simulink model "lunar_lander_sim_PWPF_2023a"  (R2023a)
settings: Solver=FixedStepAuto  StartTime=0  StopTime=250  FixedStep=0.001  RelTol=1e-3
values from neighbouring files (symbols this model uses):
  D = 0:0.01:0.9    [limit_cycle_est.m]
undefined symbols (not defined in the file or in its folder): aMode
libraries: simulink_extras x8, slpidlib x6, shared6dofsys x2, sharedutil x2
settings Model: Creator=cnsl  LastModifiedBy=s3928

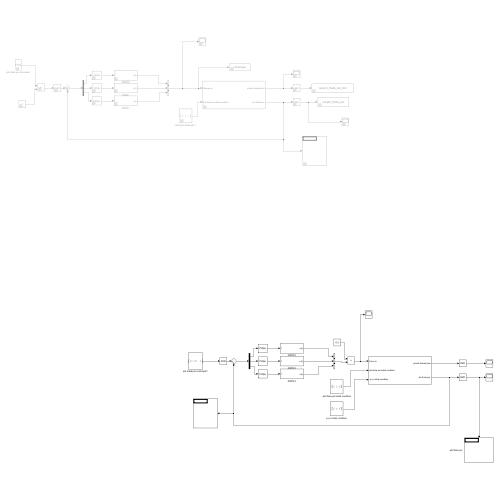
[thumbnail: Simulink's stored preview of the top-level diagram]
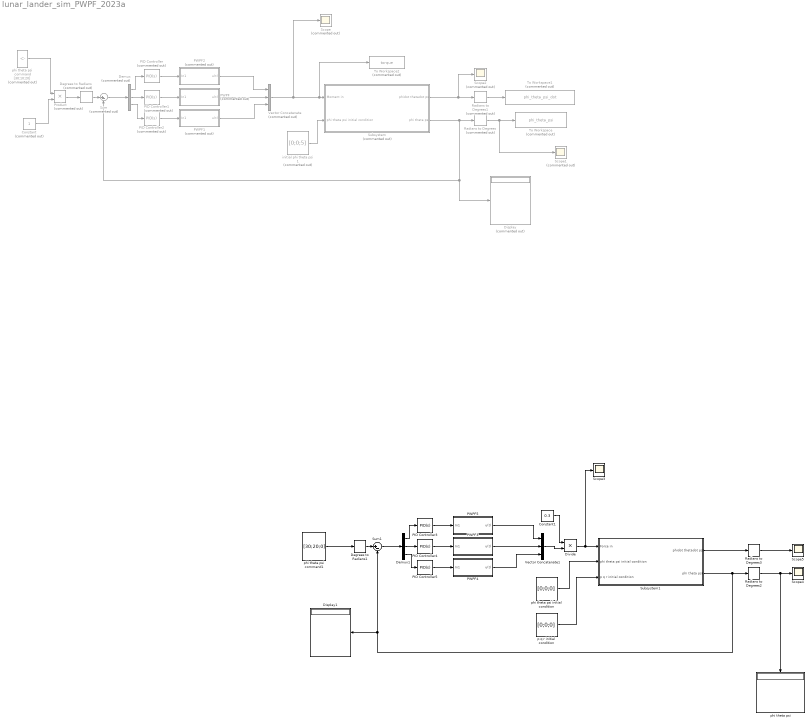
== system lunar_lander_sim_PWPF_2023a ==
  " phi theta psi initial condition" : Constant  Value=[0;0;0]
  Constant : Constant  Commented=on
  Constant1 : Constant  Value=0.3
  Degrees to Radians : simulink_extras/Transformations/Degrees to Radians  Commented=on
  Degrees to Radians1 : simulink_extras/Transformations/Degrees to Radians
  Demux : Demux  Commented=on  Outputs=3
  Demux1 : Demux  Outputs=3
  Display : Display  Commented=on
  Display1 : Display
  Divide : Product  Inputs=**
  PID Controller : slpidlib/PID Controller  Commented=on  Controller=PID  Form=Parallel  TimeDomain=Continuous-time  UseExternalTs=off  SampleTime=-1  IntegratorMethod=Forward Euler  FilterMethod=Forward Euler  ControllerParametersSource=internal  P=0  I=0  UseKiTs=off  D=0.602856201134272  N=5.45397025421619  UseFilter=on  TunerSelectOption=Transfer Function Based (PID Tuner App)  InitialConditionSource=internal  InitialConditionForIntegrator=0  InitialConditionForFilter=0  DifferentiatorICPrevScaledInput=0  ExternalReset=none  TrackingMode=off  Kt=1  LimitOutput=off  SatLimitsSource=internal  UpperSaturationLimit=inf  LowerSaturationLimit=-inf  LinearizeAsGain=on  AntiWindupMode=none  Kb=1  LimitIntegrator=off  UpperIntegratorSaturationLimit=inf  LowerIntegratorSaturationLimit=-inf  POutMin=[]  POutMax=[]  IOutMin=[]  IOutMax=[]  DOutMin=[]  DOutMax=[]  NOutMin=[]  NOutMax=[]  SumOutMin=[]  SumOutMax=[]  SaturationOutMin=[]  SaturationOutMax=[]  PParamMin=[]  PParamMax=[]  IParamMin=[]  IParamMax=[]  DParamMin=[]  DParamMax=[]  NParamMin=[]  NParamMax=[]  KbParamMin=[]  KbParamMax=[]  KtParamMin=[]  KtParamMax=[]  KbOutMin=[]  KbOutMax=[]  KtOutMin=[]  KtOutMax=[]  IntegratorOutMin=[]  IntegratorOutMax=[]  FilterOutMin=[]  FilterOutMax=[]  SumI1OutMin=[]  SumI1OutMax=[]  SumI2OutMin=[]  SumI2OutMax=[]  SumI3OutMin=[]  SumI3OutMax=[]  SumI4OutMin=[]  SumI4OutMax=[]  SumDOutMin=[]  SumDOutMax=[]  DifferentiatorOutMin=[]  DifferentiatorOutMax=[]  FilterDiffOutCoefMin=[]  FilterDiffOutCoefMax=[]  ReciprocalOutMin=[]  ReciprocalOutMax=[]  SumDenOutMin=[]  SumDenOutMax=[]  SumNumOutMin=[]  SumNumOutMax=[]  DivideOutMin=[]  DivideOutMax=[]  UdiffTsProdOutMin=[]  UdiffTsProdOutMax=[]  NTsProdOutMin=[]  NTsProdOutMax=[]  UintegralTsProdOutMin=[]  UintegralTsProdOutMax=[]  UngainTsProdOutMin=[]  UngainTsProdOutMax=[]  ClampingZeroOutDataTypeStr=Inherit: Inherit via back propagation  ClampingZeroOutMin=[]  ClampingZeroOutMax=[]  FilterDenConstantOutDataTypeStr=Inherit: Inherit via back propagation  FilterDenConstantOutMin=[]  FilterDenConstantOutMax=[]  PCopyOutDataTypeStr=Inherit: Inherit via back propagation  PCopyOutMin=[]  PCopyOutMax=[]  NCopyOutDataTypeStr=Inherit: Inherit via back propagation  NCopyOutMin=[]  NCopyOutMax=[]  IntegratorContinuousStateAttributes=''  IntegratorStateMustResolveToSignalObject=off  IntegratorRTWStateStorageClass=Auto  FilterContinuousStateAttributes=''  FilterStateMustResolveToSignalObject=off  FilterRTWStateStorageClass=Auto  ParallelPVariant=InternalParameters  IdealPVariant=Disabled  IVariant=InternalParameters  DVariant=InternalParameters  IntegratorVariant=Continuous  SatVariant=Disabled  AWVariant=Passthrough  PCopyVariant=Disabled  TRVariant=Disabled  FdbkBlocksVariant=Forward  IdealPFdbkVariant=Disabled  SatFdbkVariant=Disabled  DerivativeFilterVariant=ContFilter  NVariant=InternalParameters  NCopyVariant=Disabled  FilterICVariant=InternalICsFilter  IntegratorICVariant=InternalICs  ExternalResetVariant=Disabled  TRSumVariant=Passthrough  SumFdbkVariant=Disabled  SumVariant=Sum_PID  TsampFilterVariant=InternalTs  TsampNgainVariant=Passthrough  TsampIntegralVariant=Disabled_SignalSpec  ExternalSaturationOutDataTypeStr=Inherit: Same as second input
  PID Controller1 : slpidlib/PID Controller  Commented=on  Controller=PID  Form=Parallel  TimeDomain=Continuous-time  UseExternalTs=off  SampleTime=-1  IntegratorMethod=Forward Euler  FilterMethod=Forward Euler  ControllerParametersSource=internal  P=0.227642776770386  I=0  UseKiTs=off  D=1.19402712343922  N=5.45397025421619  UseFilter=on  TunerSelectOption=Transfer Function Based (PID Tuner App)  InitialConditionSource=internal  InitialConditionForIntegrator=0  InitialConditionForFilter=0  DifferentiatorICPrevScaledInput=0  ExternalReset=none  TrackingMode=off  Kt=1  LimitOutput=off  SatLimitsSource=internal  UpperSaturationLimit=inf  LowerSaturationLimit=-inf  LinearizeAsGain=on  AntiWindupMode=none  Kb=1  LimitIntegrator=off  UpperIntegratorSaturationLimit=inf  LowerIntegratorSaturationLimit=-inf  POutMin=[]  POutMax=[]  IOutMin=[]  IOutMax=[]  DOutMin=[]  DOutMax=[]  NOutMin=[]  NOutMax=[]  SumOutMin=[]  SumOutMax=[]  SaturationOutMin=[]  SaturationOutMax=[]  PParamMin=[]  PParamMax=[]  IParamMin=[]  IParamMax=[]  DParamMin=[]  DParamMax=[]  NParamMin=[]  NParamMax=[]  KbParamMin=[]  KbParamMax=[]  KtParamMin=[]  KtParamMax=[]  KbOutMin=[]  KbOutMax=[]  KtOutMin=[]  KtOutMax=[]  IntegratorOutMin=[]  IntegratorOutMax=[]  FilterOutMin=[]  FilterOutMax=[]  SumI1OutMin=[]  SumI1OutMax=[]  SumI2OutMin=[]  SumI2OutMax=[]  SumI3OutMin=[]  SumI3OutMax=[]  SumI4OutMin=[]  SumI4OutMax=[]  SumDOutMin=[]  SumDOutMax=[]  DifferentiatorOutMin=[]  DifferentiatorOutMax=[]  FilterDiffOutCoefMin=[]  FilterDiffOutCoefMax=[]  ReciprocalOutMin=[]  ReciprocalOutMax=[]  SumDenOutMin=[]  SumDenOutMax=[]  SumNumOutMin=[]  SumNumOutMax=[]  DivideOutMin=[]  DivideOutMax=[]  UdiffTsProdOutMin=[]  UdiffTsProdOutMax=[]  NTsProdOutMin=[]  NTsProdOutMax=[]  UintegralTsProdOutMin=[]  UintegralTsProdOutMax=[]  UngainTsProdOutMin=[]  UngainTsProdOutMax=[]  ClampingZeroOutDataTypeStr=Inherit: Inherit via back propagation  ClampingZeroOutMin=[]  ClampingZeroOutMax=[]  FilterDenConstantOutDataTypeStr=Inherit: Inherit via back propagation  FilterDenConstantOutMin=[]  FilterDenConstantOutMax=[]  PCopyOutDataTypeStr=Inherit: Inherit via back propagation  PCopyOutMin=[]  PCopyOutMax=[]  NCopyOutDataTypeStr=Inherit: Inherit via back propagation  NCopyOutMin=[]  NCopyOutMax=[]  IntegratorContinuousStateAttributes=''  IntegratorStateMustResolveToSignalObject=off  IntegratorRTWStateStorageClass=Auto  FilterContinuousStateAttributes=''  FilterStateMustResolveToSignalObject=off  FilterRTWStateStorageClass=Auto  ParallelPVariant=InternalParameters  IdealPVariant=Disabled  IVariant=InternalParameters  DVariant=InternalParameters  IntegratorVariant=Continuous  SatVariant=Disabled  AWVariant=Passthrough  PCopyVariant=Disabled  TRVariant=Disabled  FdbkBlocksVariant=Forward  IdealPFdbkVariant=Disabled  SatFdbkVariant=Disabled  DerivativeFilterVariant=ContFilter  NVariant=InternalParameters  NCopyVariant=Disabled  FilterICVariant=InternalICsFilter  IntegratorICVariant=InternalICs  ExternalResetVariant=Disabled  TRSumVariant=Passthrough  SumFdbkVariant=Disabled  SumVariant=Sum_PID  TsampFilterVariant=InternalTs  TsampNgainVariant=Passthrough  TsampIntegralVariant=Disabled_SignalSpec  ExternalSaturationOutDataTypeStr=Inherit: Same as second input
  PID Controller2 : slpidlib/PID Controller  Commented=on  Controller=PID  Form=Parallel  TimeDomain=Continuous-time  UseExternalTs=off  SampleTime=-1  IntegratorMethod=Forward Euler  FilterMethod=Forward Euler  ControllerParametersSource=internal  P=0.227642776770386  I=0  UseKiTs=off  D=1.19402712343922  N=5.45397025421619  UseFilter=on  TunerSelectOption=Transfer Function Based (PID Tuner App)  InitialConditionSource=internal  InitialConditionForIntegrator=0  InitialConditionForFilter=0  DifferentiatorICPrevScaledInput=0  ExternalReset=none  TrackingMode=off  Kt=1  LimitOutput=off  SatLimitsSource=internal  UpperSaturationLimit=inf  LowerSaturationLimit=-inf  LinearizeAsGain=on  AntiWindupMode=none  Kb=1  LimitIntegrator=off  UpperIntegratorSaturationLimit=inf  LowerIntegratorSaturationLimit=-inf  POutMin=[]  POutMax=[]  IOutMin=[]  IOutMax=[]  DOutMin=[]  DOutMax=[]  NOutMin=[]  NOutMax=[]  SumOutMin=[]  SumOutMax=[]  SaturationOutMin=[]  SaturationOutMax=[]  PParamMin=[]  PParamMax=[]  IParamMin=[]  IParamMax=[]  DParamMin=[]  DParamMax=[]  NParamMin=[]  NParamMax=[]  KbParamMin=[]  KbParamMax=[]  KtParamMin=[]  KtParamMax=[]  KbOutMin=[]  KbOutMax=[]  KtOutMin=[]  KtOutMax=[]  IntegratorOutMin=[]  IntegratorOutMax=[]  FilterOutMin=[]  FilterOutMax=[]  SumI1OutMin=[]  SumI1OutMax=[]  SumI2OutMin=[]  SumI2OutMax=[]  SumI3OutMin=[]  SumI3OutMax=[]  SumI4OutMin=[]  SumI4OutMax=[]  SumDOutMin=[]  SumDOutMax=[]  DifferentiatorOutMin=[]  DifferentiatorOutMax=[]  FilterDiffOutCoefMin=[]  FilterDiffOutCoefMax=[]  ReciprocalOutMin=[]  ReciprocalOutMax=[]  SumDenOutMin=[]  SumDenOutMax=[]  SumNumOutMin=[]  SumNumOutMax=[]  DivideOutMin=[]  DivideOutMax=[]  UdiffTsProdOutMin=[]  UdiffTsProdOutMax=[]  NTsProdOutMin=[]  NTsProdOutMax=[]  UintegralTsProdOutMin=[]  UintegralTsProdOutMax=[]  UngainTsProdOutMin=[]  UngainTsProdOutMax=[]  ClampingZeroOutDataTypeStr=Inherit: Inherit via back propagation  ClampingZeroOutMin=[]  ClampingZeroOutMax=[]  FilterDenConstantOutDataTypeStr=Inherit: Inherit via back propagation  FilterDenConstantOutMin=[]  FilterDenConstantOutMax=[]  PCopyOutDataTypeStr=Inherit: Inherit via back propagation  PCopyOutMin=[]  PCopyOutMax=[]  NCopyOutDataTypeStr=Inherit: Inherit via back propagation  NCopyOutMin=[]  NCopyOutMax=[]  IntegratorContinuousStateAttributes=''  IntegratorStateMustResolveToSignalObject=off  IntegratorRTWStateStorageClass=Auto  FilterContinuousStateAttributes=''  FilterStateMustResolveToSignalObject=off  FilterRTWStateStorageClass=Auto  ParallelPVariant=InternalParameters  IdealPVariant=Disabled  IVariant=InternalParameters  DVariant=InternalParameters  IntegratorVariant=Continuous  SatVariant=Disabled  AWVariant=Passthrough  PCopyVariant=Disabled  TRVariant=Disabled  FdbkBlocksVariant=Forward  IdealPFdbkVariant=Disabled  SatFdbkVariant=Disabled  DerivativeFilterVariant=ContFilter  NVariant=InternalParameters  NCopyVariant=Disabled  FilterICVariant=InternalICsFilter  IntegratorICVariant=InternalICs  ExternalResetVariant=Disabled  TRSumVariant=Passthrough  SumFdbkVariant=Disabled  SumVariant=Sum_PID  TsampFilterVariant=InternalTs  TsampNgainVariant=Passthrough  TsampIntegralVariant=Disabled_SignalSpec  ExternalSaturationOutDataTypeStr=Inherit: Same as second input
  PID Controller3 : slpidlib/PID Controller  Controller=PID  Form=Parallel  TimeDomain=Continuous-time  UseExternalTs=off  SampleTime=-1  IntegratorMethod=Forward Euler  FilterMethod=Forward Euler  ControllerParametersSource=internal  P=3  I=0.5  UseKiTs=off  D=8  N=1000  UseFilter=on  TunerSelectOption=Transfer Function Based (PID Tuner App)  InitialConditionSource=internal  InitialConditionForIntegrator=0  InitialConditionForFilter=0  DifferentiatorICPrevScaledInput=0  ExternalReset=none  TrackingMode=off  Kt=1  LimitOutput=off  SatLimitsSource=internal  UpperSaturationLimit=inf  LowerSaturationLimit=-inf  LinearizeAsGain=on  AntiWindupMode=none  Kb=1  LimitIntegrator=off  UpperIntegratorSaturationLimit=inf  LowerIntegratorSaturationLimit=-inf  POutMin=[]  POutMax=[]  IOutMin=[]  IOutMax=[]  DOutMin=[]  DOutMax=[]  NOutMin=[]  NOutMax=[]  SumOutMin=[]  SumOutMax=[]  SaturationOutMin=[]  SaturationOutMax=[]  PParamMin=[]  PParamMax=[]  IParamMin=[]  IParamMax=[]  DParamMin=[]  DParamMax=[]  NParamMin=[]  NParamMax=[]  KbParamMin=[]  KbParamMax=[]  KtParamMin=[]  KtParamMax=[]  KbOutMin=[]  KbOutMax=[]  KtOutMin=[]  KtOutMax=[]  IntegratorOutMin=[]  IntegratorOutMax=[]  FilterOutMin=[]  FilterOutMax=[]  SumI1OutMin=[]  SumI1OutMax=[]  SumI2OutMin=[]  SumI2OutMax=[]  SumI3OutMin=[]  SumI3OutMax=[]  SumI4OutMin=[]  SumI4OutMax=[]  SumDOutMin=[]  SumDOutMax=[]  DifferentiatorOutMin=[]  DifferentiatorOutMax=[]  FilterDiffOutCoefMin=[]  FilterDiffOutCoefMax=[]  ReciprocalOutMin=[]  ReciprocalOutMax=[]  SumDenOutMin=[]  SumDenOutMax=[]  SumNumOutMin=[]  SumNumOutMax=[]  DivideOutMin=[]  DivideOutMax=[]  UdiffTsProdOutMin=[]  UdiffTsProdOutMax=[]  NTsProdOutMin=[]  NTsProdOutMax=[]  UintegralTsProdOutMin=[]  UintegralTsProdOutMax=[]  UngainTsProdOutMin=[]  UngainTsProdOutMax=[]  ClampingZeroOutDataTypeStr=Inherit: Inherit via back propagation  ClampingZeroOutMin=[]  ClampingZeroOutMax=[]  FilterDenConstantOutDataTypeStr=Inherit: Inherit via back propagation  FilterDenConstantOutMin=[]  FilterDenConstantOutMax=[]  PCopyOutDataTypeStr=Inherit: Inherit via back propagation  PCopyOutMin=[]  PCopyOutMax=[]  NCopyOutDataTypeStr=Inherit: Inherit via back propagation  NCopyOutMin=[]  NCopyOutMax=[]  IntegratorContinuousStateAttributes=''  IntegratorStateMustResolveToSignalObject=off  IntegratorRTWStateStorageClass=Auto  FilterContinuousStateAttributes=''  FilterStateMustResolveToSignalObject=off  FilterRTWStateStorageClass=Auto  ParallelPVariant=InternalParameters  IdealPVariant=Disabled  IVariant=InternalParameters  DVariant=InternalParameters  IntegratorVariant=Continuous  SatVariant=Disabled  AWVariant=Passthrough  PCopyVariant=Disabled  TRVariant=Disabled  FdbkBlocksVariant=Forward  IdealPFdbkVariant=Disabled  SatFdbkVariant=Disabled  DerivativeFilterVariant=ContFilter  NVariant=InternalParameters  NCopyVariant=Disabled  FilterICVariant=InternalICsFilter  IntegratorICVariant=InternalICs  ExternalResetVariant=Disabled  TRSumVariant=Passthrough  SumFdbkVariant=Disabled  SumVariant=Sum_PID  TsampFilterVariant=InternalTs  TsampNgainVariant=Passthrough  TsampIntegralVariant=Disabled_SignalSpec  ExternalSaturationOutDataTypeStr=Inherit: Same as second input
  PID Controller4 : slpidlib/PID Controller  Controller=PID  Form=Parallel  TimeDomain=Continuous-time  UseExternalTs=off  SampleTime=-1  IntegratorMethod=Forward Euler  FilterMethod=Forward Euler  ControllerParametersSource=internal  P=2  I=0.1  UseKiTs=off  D=8  N=1000  UseFilter=on  TunerSelectOption=Transfer Function Based (PID Tuner App)  InitialConditionSource=internal  InitialConditionForIntegrator=0  InitialConditionForFilter=0  DifferentiatorICPrevScaledInput=0  ExternalReset=none  TrackingMode=off  Kt=1  LimitOutput=off  SatLimitsSource=internal  UpperSaturationLimit=inf  LowerSaturationLimit=-inf  LinearizeAsGain=on  AntiWindupMode=none  Kb=1  LimitIntegrator=off  UpperIntegratorSaturationLimit=inf  LowerIntegratorSaturationLimit=-inf  POutMin=[]  POutMax=[]  IOutMin=[]  IOutMax=[]  DOutMin=[]  DOutMax=[]  NOutMin=[]  NOutMax=[]  SumOutMin=[]  SumOutMax=[]  SaturationOutMin=[]  SaturationOutMax=[]  PParamMin=[]  PParamMax=[]  IParamMin=[]  IParamMax=[]  DParamMin=[]  DParamMax=[]  NParamMin=[]  NParamMax=[]  KbParamMin=[]  KbParamMax=[]  KtParamMin=[]  KtParamMax=[]  KbOutMin=[]  KbOutMax=[]  KtOutMin=[]  KtOutMax=[]  IntegratorOutMin=[]  IntegratorOutMax=[]  FilterOutMin=[]  FilterOutMax=[]  SumI1OutMin=[]  SumI1OutMax=[]  SumI2OutMin=[]  SumI2OutMax=[]  SumI3OutMin=[]  SumI3OutMax=[]  SumI4OutMin=[]  SumI4OutMax=[]  SumDOutMin=[]  SumDOutMax=[]  DifferentiatorOutMin=[]  DifferentiatorOutMax=[]  FilterDiffOutCoefMin=[]  FilterDiffOutCoefMax=[]  ReciprocalOutMin=[]  ReciprocalOutMax=[]  SumDenOutMin=[]  SumDenOutMax=[]  SumNumOutMin=[]  SumNumOutMax=[]  DivideOutMin=[]  DivideOutMax=[]  UdiffTsProdOutMin=[]  UdiffTsProdOutMax=[]  NTsProdOutMin=[]  NTsProdOutMax=[]  UintegralTsProdOutMin=[]  UintegralTsProdOutMax=[]  UngainTsProdOutMin=[]  UngainTsProdOutMax=[]  ClampingZeroOutDataTypeStr=Inherit: Inherit via back propagation  ClampingZeroOutMin=[]  ClampingZeroOutMax=[]  FilterDenConstantOutDataTypeStr=Inherit: Inherit via back propagation  FilterDenConstantOutMin=[]  FilterDenConstantOutMax=[]  PCopyOutDataTypeStr=Inherit: Inherit via back propagation  PCopyOutMin=[]  PCopyOutMax=[]  NCopyOutDataTypeStr=Inherit: Inherit via back propagation  NCopyOutMin=[]  NCopyOutMax=[]  IntegratorContinuousStateAttributes=''  IntegratorStateMustResolveToSignalObject=off  IntegratorRTWStateStorageClass=Auto  FilterContinuousStateAttributes=''  FilterStateMustResolveToSignalObject=off  FilterRTWStateStorageClass=Auto  ParallelPVariant=InternalParameters  IdealPVariant=Disabled  IVariant=InternalParameters  DVariant=InternalParameters  IntegratorVariant=Continuous  SatVariant=Disabled  AWVariant=Passthrough  PCopyVariant=Disabled  TRVariant=Disabled  FdbkBlocksVariant=Forward  IdealPFdbkVariant=Disabled  SatFdbkVariant=Disabled  DerivativeFilterVariant=ContFilter  NVariant=InternalParameters  NCopyVariant=Disabled  FilterICVariant=InternalICsFilter  IntegratorICVariant=InternalICs  ExternalResetVariant=Disabled  TRSumVariant=Passthrough  SumFdbkVariant=Disabled  SumVariant=Sum_PID  TsampFilterVariant=InternalTs  TsampNgainVariant=Passthrough  TsampIntegralVariant=Disabled_SignalSpec  ExternalSaturationOutDataTypeStr=Inherit: Same as second input
  PID Controller5 : slpidlib/PID Controller  Controller=PID  Form=Parallel  TimeDomain=Continuous-time  UseExternalTs=off  SampleTime=-1  IntegratorMethod=Forward Euler  FilterMethod=Forward Euler  ControllerParametersSource=internal  P=3  I=0.2  UseKiTs=off  D=12  N=1000  UseFilter=on  TunerSelectOption=Transfer Function Based (PID Tuner App)  InitialConditionSource=internal  InitialConditionForIntegrator=0  InitialConditionForFilter=0  DifferentiatorICPrevScaledInput=0  ExternalReset=none  TrackingMode=off  Kt=1  LimitOutput=off  SatLimitsSource=internal  UpperSaturationLimit=inf  LowerSaturationLimit=-inf  LinearizeAsGain=on  AntiWindupMode=none  Kb=1  LimitIntegrator=off  UpperIntegratorSaturationLimit=inf  LowerIntegratorSaturationLimit=-inf  POutMin=[]  POutMax=[]  IOutMin=[]  IOutMax=[]  DOutMin=[]  DOutMax=[]  NOutMin=[]  NOutMax=[]  SumOutMin=[]  SumOutMax=[]  SaturationOutMin=[]  SaturationOutMax=[]  PParamMin=[]  PParamMax=[]  IParamMin=[]  IParamMax=[]  DParamMin=[]  DParamMax=[]  NParamMin=[]  NParamMax=[]  KbParamMin=[]  KbParamMax=[]  KtParamMin=[]  KtParamMax=[]  KbOutMin=[]  KbOutMax=[]  KtOutMin=[]  KtOutMax=[]  IntegratorOutMin=[]  IntegratorOutMax=[]  FilterOutMin=[]  FilterOutMax=[]  SumI1OutMin=[]  SumI1OutMax=[]  SumI2OutMin=[]  SumI2OutMax=[]  SumI3OutMin=[]  SumI3OutMax=[]  SumI4OutMin=[]  SumI4OutMax=[]  SumDOutMin=[]  SumDOutMax=[]  DifferentiatorOutMin=[]  DifferentiatorOutMax=[]  FilterDiffOutCoefMin=[]  FilterDiffOutCoefMax=[]  ReciprocalOutMin=[]  ReciprocalOutMax=[]  SumDenOutMin=[]  SumDenOutMax=[]  SumNumOutMin=[]  SumNumOutMax=[]  DivideOutMin=[]  DivideOutMax=[]  UdiffTsProdOutMin=[]  UdiffTsProdOutMax=[]  NTsProdOutMin=[]  NTsProdOutMax=[]  UintegralTsProdOutMin=[]  UintegralTsProdOutMax=[]  UngainTsProdOutMin=[]  UngainTsProdOutMax=[]  ClampingZeroOutDataTypeStr=Inherit: Inherit via back propagation  ClampingZeroOutMin=[]  ClampingZeroOutMax=[]  FilterDenConstantOutDataTypeStr=Inherit: Inherit via back propagation  FilterDenConstantOutMin=[]  FilterDenConstantOutMax=[]  PCopyOutDataTypeStr=Inherit: Inherit via back propagation  PCopyOutMin=[]  PCopyOutMax=[]  NCopyOutDataTypeStr=Inherit: Inherit via back propagation  NCopyOutMin=[]  NCopyOutMax=[]  IntegratorContinuousStateAttributes=''  IntegratorStateMustResolveToSignalObject=off  IntegratorRTWStateStorageClass=Auto  FilterContinuousStateAttributes=''  FilterStateMustResolveToSignalObject=off  FilterRTWStateStorageClass=Auto  ParallelPVariant=InternalParameters  IdealPVariant=Disabled  IVariant=InternalParameters  DVariant=InternalParameters  IntegratorVariant=Continuous  SatVariant=Disabled  AWVariant=Passthrough  PCopyVariant=Disabled  TRVariant=Disabled  FdbkBlocksVariant=Forward  IdealPFdbkVariant=Disabled  SatFdbkVariant=Disabled  DerivativeFilterVariant=ContFilter  NVariant=InternalParameters  NCopyVariant=Disabled  FilterICVariant=InternalICsFilter  IntegratorICVariant=InternalICs  ExternalResetVariant=Disabled  TRSumVariant=Passthrough  SumFdbkVariant=Disabled  SumVariant=Sum_PID  TsampFilterVariant=InternalTs  TsampNgainVariant=Passthrough  TsampIntegralVariant=Disabled_SignalSpec  ExternalSaturationOutDataTypeStr=Inherit: Same as second input
  PWPF : Subsystem  Commented=on
  PWPF1 : Subsystem  Commented=on
  PWPF2 : Subsystem  Commented=on
  PWPF3 : Subsystem
  PWPF4 : Subsystem
  PWPF5 : Subsystem
  Product : Product  Commented=on
  Radians to Degrees : simulink_extras/Transformations/Radians to Degrees  Commented=on
  Radians to Degrees1 : simulink_extras/Transformations/Radians to Degrees  Commented=on
  Radians to Degrees2 : simulink_extras/Transformations/Radians to Degrees
  Radians to Degrees3 : simulink_extras/Transformations/Radians to Degrees
  Scope : Scope  Commented=on
  Scope1 : Scope  Commented=on
  Scope2 : Scope  Commented=on
  Scope3 : Scope
  Scope4 : Scope
  Scope5 : Scope
  Subsystem : Subsystem  Commented=on
  Subsystem1 : Subsystem
  Sum : Sum  Commented=on  Inputs=|+-
  Sum1 : Sum  Inputs=|+-
  To Workspace : ToWorkspace  Commented=on  VariableName=phi_theta_psi  SaveFormat=Timeseries  SampleTime=-1
  To Workspace1 : ToWorkspace  Commented=on  VariableName=phi_theta_psi_dot  SaveFormat=Timeseries  SampleTime=-1
  To Workspace2 : ToWorkspace  Commented=on  VariableName=torque  SaveFormat=Timeseries  SampleTime=-1
  Vector Concatenate : Concatenate  Commented=on  NumInputs=3
  Vector Concatenate1 : Concatenate  NumInputs=3
  initial phi theta psi 1 : Constant  Commented=on  Value=[0;0;5]
  p q r initial condition : Constant  Value=[0;0;0]
  "phi theta psi " : Display
  phi theta psi command : Constant  Commented=on  Value=[30;10;20]
  phi theta psi command1 : Constant  Value=[30;20;0]
  wires:
  Subsystem/2("phi theta psi ") -> Radians to Degrees/1, Display/1, Sum/2
  Degrees to Radians/1 -> Sum/1
  Radians to Degrees/1 -> Scope1/1, To Workspace/1
  Vector Concatenate/1 -> Scope/1, Subsystem/1(Moment in), To Workspace2/1
  initial phi theta psi 1/1 -> Subsystem/2("phi theta psi initial condition ")
  phi theta psi command/1 -> Product/1
  Product/1 -> Degrees to Radians/1
  Constant/1 -> Product/2
  Demux/1 -> PID Controller/1
  Demux/3 -> PID Controller2/1
  PID Controller2/1 -> PWPF1/1(In1)
  Subsystem/1(phidot thetadot psi) -> Scope2/1, Radians to Degrees1/1
  Sum/1 -> Demux/1
  Radians to Degrees1/1 -> To Workspace1/1
  PID Controller/1 -> PWPF2/1(In1)
  Demux/2 -> PID Controller1/1
  PWPF/1(u(t)) -> Vector Concatenate/2
  PID Controller1/1 -> PWPF/1(In1)
  PWPF1/1(u(t)) -> Vector Concatenate/3
  PWPF2/1(u(t)) -> Vector Concatenate/1
  Sum1/1 -> Demux1/1
  phi theta psi command1/1 -> Degrees to Radians1/1
  Demux1/2 -> PID Controller4/1
  Demux1/3 -> PID Controller5/1
  Subsystem1/1(phidot thetadot psi) -> Radians to Degrees3/1
  Demux1/1 -> PID Controller3/1
  Degrees to Radians1/1 -> Sum1/1
  Radians to Degrees2/1 -> Scope4/1, "phi theta psi "/1
  " phi theta psi initial condition"/1 -> Subsystem1/2("phi theta psi initial condition ")
  Subsystem1/2("phi theta psi ") -> Radians to Degrees2/1, Sum1/2, Display1/1
  PID Controller3/1 -> PWPF5/1(In1)
  PID Controller5/1 -> PWPF4/1(In1)
  PID Controller4/1 -> PWPF3/1(In1)
  Radians to Degrees3/1 -> Scope5/1
  p q r initial condition/1 -> Subsystem1/3(" p q r initial condition")
  PWPF3/1(u(t)) -> Vector Concatenate1/2
  PWPF4/1(u(t)) -> Vector Concatenate1/3
  PWPF5/1(u(t)) -> Vector Concatenate1/1
  Vector Concatenate1/1 -> Divide/2
  Divide/1 -> Scope3/1, Subsystem1/1(Force in)
  Constant1/1 -> Divide/1

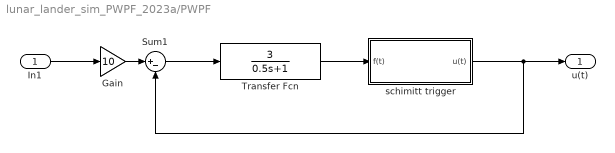
== system lunar_lander_sim_PWPF_2023a/PWPF ==
  In1 : Inport
  Gain : Gain  Gain=10
  Sum1 : Sum  Inputs=|+-
  Transfer Fcn : TransferFcn  Numerator=[3]  Denominator=[0.5 1]
  schimitt trigger : Subsystem
  u(t) : Outport
  wires:
  schimitt trigger/1(u(t)) -> u(t)/1, Sum1/2
  Gain/1 -> Sum1/1
  Sum1/1 -> Transfer Fcn/1
  Transfer Fcn/1 -> schimitt trigger/1(f(t))
  In1/1 -> Gain/1

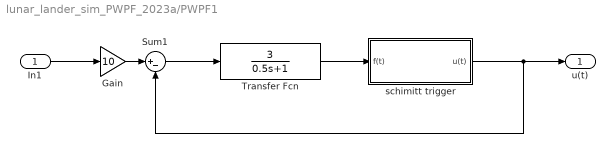
== system lunar_lander_sim_PWPF_2023a/PWPF1 ==
  In1 : Inport
  Gain : Gain  Gain=10
  Sum1 : Sum  Inputs=|+-
  Transfer Fcn : TransferFcn  Numerator=[3]  Denominator=[0.5 1]
  schimitt trigger : Subsystem
  u(t) : Outport
  wires:
  In1/1 -> Gain/1
  Transfer Fcn/1 -> schimitt trigger/1(f(t))
  Sum1/1 -> Transfer Fcn/1
  Gain/1 -> Sum1/1
  schimitt trigger/1(u(t)) -> Sum1/2, u(t)/1

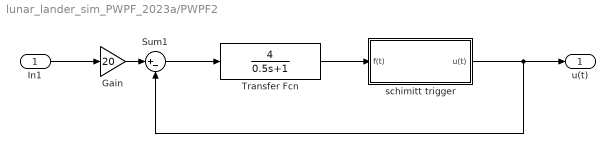
== system lunar_lander_sim_PWPF_2023a/PWPF2 ==
  In1 : Inport
  Gain : Gain  Gain=20
  Sum1 : Sum  Inputs=|+-
  Transfer Fcn : TransferFcn  Numerator=[4]  Denominator=[0.5 1]
  schimitt trigger : Subsystem
  u(t) : Outport
  wires:
  schimitt trigger/1(u(t)) -> u(t)/1, Sum1/2
  Gain/1 -> Sum1/1
  Sum1/1 -> Transfer Fcn/1
  Transfer Fcn/1 -> schimitt trigger/1(f(t))
  In1/1 -> Gain/1

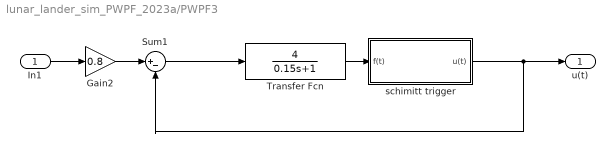
== system lunar_lander_sim_PWPF_2023a/PWPF3 ==
  In1 : Inport
  Gain2 : Gain  Gain=0.8
  Sum1 : Sum  Inputs=|+-
  Transfer Fcn : TransferFcn  Numerator=[4]  Denominator=[0.15 1]
  schimitt trigger : Subsystem
  u(t) : Outport
  wires:
  In1/1 -> Gain2/1
  Gain2/1 -> Sum1/1
  schimitt trigger/1(u(t)) -> u(t)/1, Sum1/2
  Sum1/1 -> Transfer Fcn/1
  Transfer Fcn/1 -> schimitt trigger/1(f(t))

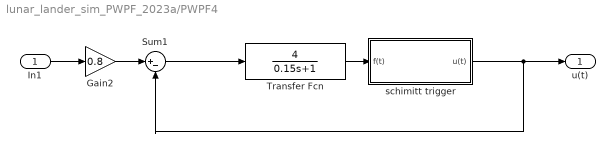
== system lunar_lander_sim_PWPF_2023a/PWPF4 ==
  In1 : Inport
  Gain2 : Gain  Gain=0.8
  Sum1 : Sum  Inputs=|+-
  Transfer Fcn : TransferFcn  Numerator=[4]  Denominator=[0.15 1]
  schimitt trigger : Subsystem
  u(t) : Outport
  wires:
  Transfer Fcn/1 -> schimitt trigger/1(f(t))
  Sum1/1 -> Transfer Fcn/1
  schimitt trigger/1(u(t)) -> Sum1/2, u(t)/1
  Gain2/1 -> Sum1/1
  In1/1 -> Gain2/1

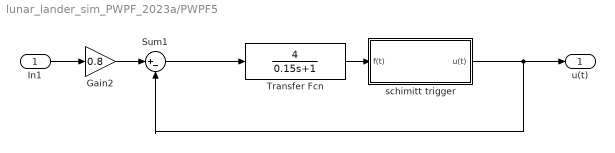
== system lunar_lander_sim_PWPF_2023a/PWPF5 ==
  In1 : Inport
  Gain2 : Gain  Gain=0.8
  Sum1 : Sum  Inputs=|+-
  Transfer Fcn : TransferFcn  Numerator=[4]  Denominator=[0.15 1]
  schimitt trigger : Subsystem
  u(t) : Outport
  wires:
  Transfer Fcn/1 -> schimitt trigger/1(f(t))
  Sum1/1 -> Transfer Fcn/1
  schimitt trigger/1(u(t)) -> Sum1/2, u(t)/1
  Gain2/1 -> Sum1/1
  In1/1 -> Gain2/1

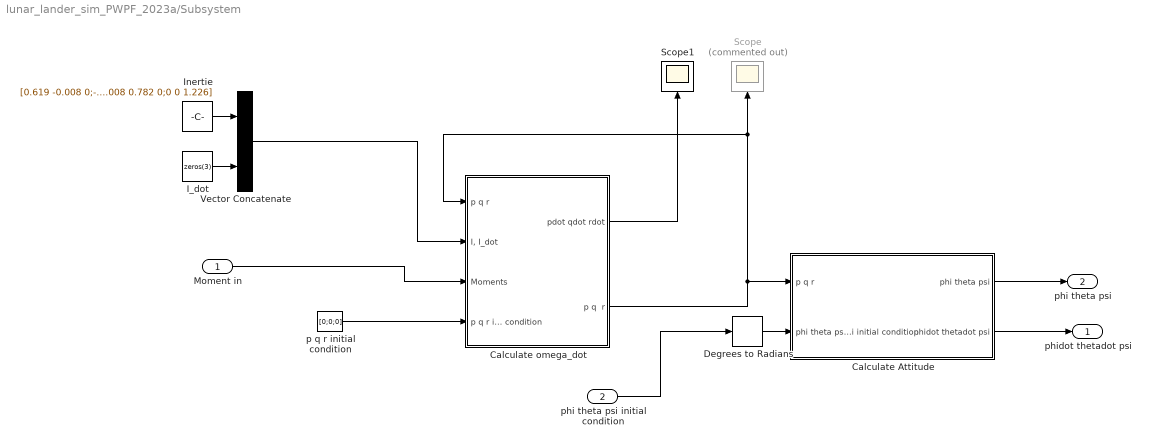
== system lunar_lander_sim_PWPF_2023a/Subsystem ==
  Moment in : Inport
  "phi theta psi initial condition " : Inport  Port=2
  " p q r initial condition" : Constant  Value=[0;0;0]
  "Calculate Attitude " : Subsystem
  Calculate omega_dot : Subsystem  AncestorBlock=shared6dofsys/Calculate omega_dot  mask{aMode=aMode}
      mask init:
      | if aerosharedtest(gcb)
      |     aerosharedicon('shared');
      | else
      |     sharedautoicon('shared');
      | end
      settings: LibrarySourceBlock=shared6dofsys/Calculate omega_dot
  Degrees to Radians : simulink_extras/Transformations/Degrees to Radians
  I_dot : Constant  Value=zeros(3)
  Inertie : Constant  Value=[0.619 -0.008 0;-0.008 0.782 0;0 0 1.226]
  Scope : Scope  Commented=on
  Scope1 : Scope
  Vector Concatenate : Concatenate  Mode=Multidimensional array
  phidot thetadot psi : Outport
  "phi theta psi " : Outport  Port=2
  wires:
  Vector Concatenate/1 -> Calculate omega_dot/2("I, I_dot")
  Inertie/1 -> Vector Concatenate/1
  Calculate omega_dot/2(p q  r) -> Scope/1, Calculate omega_dot/1(p q r), "Calculate Attitude "/1(p q r)
  I_dot/1 -> Vector Concatenate/2
  Moment in/1 -> Calculate omega_dot/3(Moments)
  " p q r initial condition"/1 -> Calculate omega_dot/4(p q r initial condition)
  "Calculate Attitude "/1("phi theta psi ") -> "phi theta psi "/1
  Degrees to Radians/1 -> "Calculate Attitude "/2("phi theta psi initial condition ")
  "phi theta psi initial condition "/1 -> Degrees to Radians/1
  "Calculate Attitude "/2(phidot thetadot psi) -> phidot thetadot psi/1
  Calculate omega_dot/1(pdot qdot rdot) -> Scope1/1

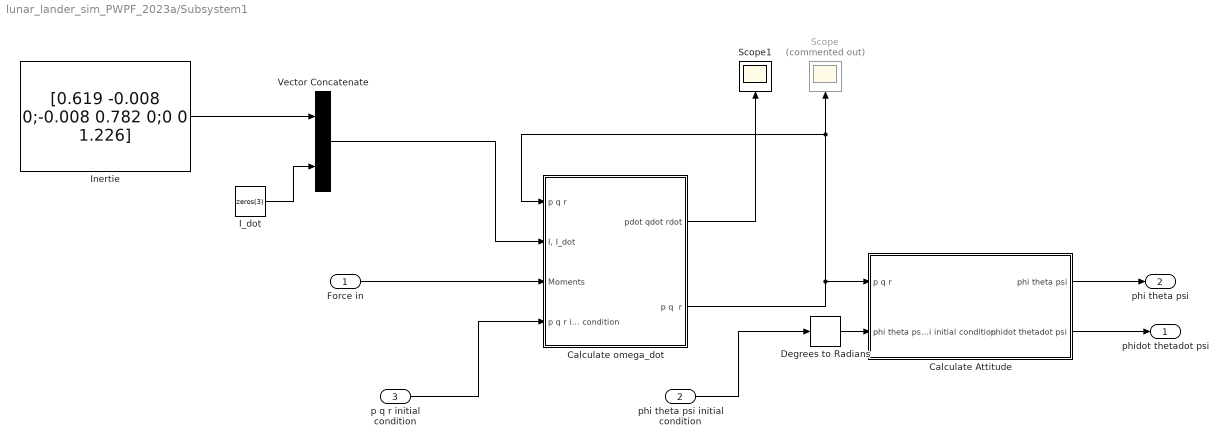
== system lunar_lander_sim_PWPF_2023a/Subsystem1 ==
  Force in : Inport
  "phi theta psi initial condition " : Inport  Port=2
  " p q r initial condition" : Inport  Port=3
  "Calculate Attitude " : Subsystem
  Calculate omega_dot : Subsystem  AncestorBlock=shared6dofsys/Calculate omega_dot  mask{aMode=aMode}
      mask init:
      | if aerosharedtest(gcb)
      |     aerosharedicon('shared');
      | else
      |     sharedautoicon('shared');
      | end
      settings: LibrarySourceBlock=shared6dofsys/Calculate omega_dot
  Degrees to Radians : simulink_extras/Transformations/Degrees to Radians
  I_dot : Constant  Value=zeros(3)
  Inertie : Constant  Value=[0.619 -0.008 0;-0.008 0.782 0;0 0 1.226]
  Scope : Scope  Commented=on
  Scope1 : Scope
  Vector Concatenate : Concatenate  Mode=Multidimensional array
  phidot thetadot psi : Outport
  "phi theta psi " : Outport  Port=2
  wires:
  Vector Concatenate/1 -> Calculate omega_dot/2("I, I_dot")
  Inertie/1 -> Vector Concatenate/1
  Calculate omega_dot/2(p q  r) -> Scope/1, Calculate omega_dot/1(p q r), "Calculate Attitude "/1(p q r)
  I_dot/1 -> Vector Concatenate/2
  " p q r initial condition"/1 -> Calculate omega_dot/4(p q r initial condition)
  "Calculate Attitude "/1("phi theta psi ") -> "phi theta psi "/1
  Degrees to Radians/1 -> "Calculate Attitude "/2("phi theta psi initial condition ")
  "phi theta psi initial condition "/1 -> Degrees to Radians/1
  "Calculate Attitude "/2(phidot thetadot psi) -> phidot thetadot psi/1
  Calculate omega_dot/1(pdot qdot rdot) -> Scope1/1
  Force in/1 -> Calculate omega_dot/3(Moments)

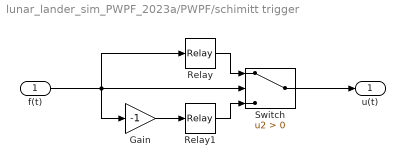
== system lunar_lander_sim_PWPF_2023a/PWPF/schimitt trigger ==
  f(t) : Inport
  Gain : Gain  Gain=-1
  Relay : Relay  OnSwitchValue=0.5  OffSwitchValue=0.15  OnOutputValue=10
  Relay1 : Relay  OnSwitchValue=0.5  OffSwitchValue=0.15  OnOutputValue=-10
  Switch : Switch  Criteria=u2 > Threshold  SaturateOnIntegerOverflow=off  InputSameDT=off
  u(t) : Outport
  wires:
  f(t)/1 -> Relay/1, Gain/1, Switch/2
  Relay1/1 -> Switch/3
  Gain/1 -> Relay1/1
  Relay/1 -> Switch/1
  Switch/1 -> u(t)/1

== system lunar_lander_sim_PWPF_2023a/PWPF1/schimitt trigger ==
  f(t) : Inport
  Gain : Gain  Gain=-1
  Relay : Relay  OnSwitchValue=0.5  OffSwitchValue=0.15  OnOutputValue=10
  Relay1 : Relay  OnSwitchValue=0.5  OffSwitchValue=0.15  OnOutputValue=-10
  Switch : Switch  Criteria=u2 > Threshold  SaturateOnIntegerOverflow=off  InputSameDT=off
  u(t) : Outport
  wires:
  Switch/1 -> u(t)/1
  Relay/1 -> Switch/1
  Gain/1 -> Relay1/1
  Relay1/1 -> Switch/3
  f(t)/1 -> Switch/2, Gain/1, Relay/1

== system lunar_lander_sim_PWPF_2023a/PWPF2/schimitt trigger ==
  f(t) : Inport
  Gain : Gain  Gain=-1
  Relay : Relay  OnSwitchValue=0.45  OffSwitchValue=0.15  OnOutputValue=10
  Relay1 : Relay  OnSwitchValue=0.45  OffSwitchValue=0.15  OnOutputValue=-10
  Switch : Switch  Criteria=u2 > Threshold  SaturateOnIntegerOverflow=off  InputSameDT=off
  u(t) : Outport
  wires:
  f(t)/1 -> Relay/1, Gain/1, Switch/2
  Relay1/1 -> Switch/3
  Gain/1 -> Relay1/1
  Relay/1 -> Switch/1
  Switch/1 -> u(t)/1

== system lunar_lander_sim_PWPF_2023a/PWPF3/schimitt trigger ==
  f(t) : Inport
  Gain : Gain  Gain=-1
  Relay : Relay  OnSwitchValue=0.5  OffSwitchValue=0.15  OnOutputValue=4.5
  Relay1 : Relay  OnSwitchValue=0.5  OffSwitchValue=0.15  OnOutputValue=-4.5
  Switch : Switch  Criteria=u2 > Threshold  SaturateOnIntegerOverflow=off  InputSameDT=off
  u(t) : Outport
  wires:
  Switch/1 -> u(t)/1
  Relay/1 -> Switch/1
  Gain/1 -> Relay1/1
  Relay1/1 -> Switch/3
  f(t)/1 -> Switch/2, Gain/1, Relay/1

== system lunar_lander_sim_PWPF_2023a/PWPF4/schimitt trigger ==
  f(t) : Inport
  Gain : Gain  Gain=-1
  Relay : Relay  OnSwitchValue=0.5  OffSwitchValue=0.15  OnOutputValue=4.5
  Relay1 : Relay  OnSwitchValue=0.5  OffSwitchValue=0.15  OnOutputValue=-4.5
  Switch : Switch  Criteria=u2 > Threshold  SaturateOnIntegerOverflow=off  InputSameDT=off
  u(t) : Outport
  wires:
  f(t)/1 -> Relay/1, Gain/1, Switch/2
  Relay1/1 -> Switch/3
  Gain/1 -> Relay1/1
  Relay/1 -> Switch/1
  Switch/1 -> u(t)/1

== system lunar_lander_sim_PWPF_2023a/PWPF5/schimitt trigger ==
  f(t) : Inport
  Gain : Gain  Gain=-1
  Relay : Relay  OnSwitchValue=0.5  OffSwitchValue=0.15  OnOutputValue=4.5
  Relay1 : Relay  OnSwitchValue=0.5  OffSwitchValue=0.15  OnOutputValue=-4.5
  Switch : Switch  Criteria=u2 > Threshold  SaturateOnIntegerOverflow=off  InputSameDT=off
  u(t) : Outport
  wires:
  f(t)/1 -> Relay/1, Gain/1, Switch/2
  Relay1/1 -> Switch/3
  Gain/1 -> Relay1/1
  Relay/1 -> Switch/1
  Switch/1 -> u(t)/1

== system lunar_lander_sim_PWPF_2023a/Subsystem/Calculate Attitude  ==
  p q r : Inport
  "phi theta psi initial condition " : Inport  Port=2
  " " : Integrator  InitialConditionSource=external
  phidot thetadot psidot : shared6dofsys/DCM & Euler Angles (Euler)/phidot thetadot psidot  SystemSampleTime=-1  VariantActivationTime=update diagram  Latency=0  AutoFrameSizeCalculation=off
  "phi theta psi " : Outport
  phidot thetadot psi : Outport  Port=2
  wires:
  "phi theta psi initial condition "/1 -> " "/2
  " "/1 -> phidot thetadot psidot/2, "phi theta psi "/1
  phidot thetadot psidot/1 -> phidot thetadot psi/1, " "/1
  p q r/1 -> phidot thetadot psidot/1

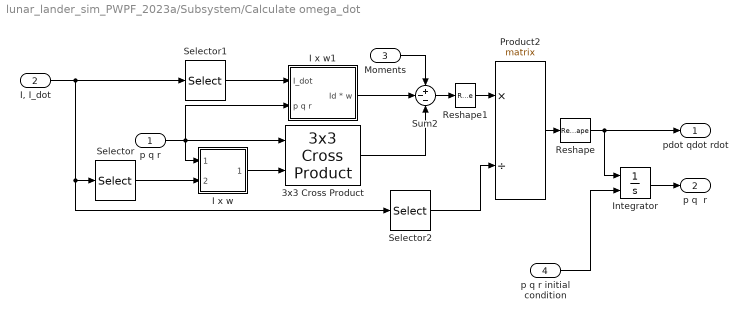
== system lunar_lander_sim_PWPF_2023a/Subsystem/Calculate omega_dot ==
  p q r : Inport  OutDataTypeStr=double
  "I, I_dot" : Inport  Port=2  OutDataTypeStr=double
  Moments : Inport  Port=3  OutDataTypeStr=double
  p q r initial condition : Inport  Port=4
  3x3 Cross Product : sharedutil/3x3 Cross Product  aMode=aMode
  I x w : Subsystem
  I x w1 : Subsystem
  Integrator : Integrator  InitialConditionSource=external
  Product2 : Product  Inputs=*/  Multiplication=Matrix(*)  SaturateOnIntegerOverflow=on  OutDataTypeStr=Inherit: Same as first input
  Reshape : Reshape
  Reshape1 : Reshape  OutputDimensionality=Row vector (2-D)
  Selector : Selector  NumberOfDimensions=2  InputPortWidth=2  IndexOptions=Index vector (dialog),Select all  Indices=1:3,-1  OutputSizes=1
  Selector1 : Selector  NumberOfDimensions=2  InputPortWidth=2  IndexOptions=Index vector (dialog),Select all  Indices=4:6,-1  OutputSizes=1
  Selector2 : Selector  NumberOfDimensions=2  InputPortWidth=2  IndexOptions=Index vector (dialog),Select all  Indices=1:3,-1  OutputSizes=1
  Sum2 : Sum  Inputs=+--  SaturateOnIntegerOverflow=on
  pdot qdot rdot : Outport  OutDataTypeStr=double  VectorParamsAs1DForOutWhenUnconnected=off
  p q  r : Outport  Port=2
  wires:
  p q r initial condition/1 -> Integrator/2
  Integrator/1 -> p q  r/1
  Reshape/1 -> pdot qdot rdot/1, Integrator/1
  Selector/1 -> I x w/2(Inertia)
  Selector2/1 -> Product2/2
  "I, I_dot"/1 -> Selector/1, Selector2/1, Selector1/1
  p q r/1 -> 3x3 Cross Product/1, I x w1/2(p q r), I x w/1(p q r)
  Product2/1 -> Reshape/1
  Sum2/1 -> Reshape1/1
  Moments/1 -> Sum2/1
  I x w1/1(Id * w) -> Sum2/2
  Selector1/1 -> I x w1/1(I_dot)
  I x w/1(I * w) -> 3x3 Cross Product/2
  Reshape1/1 -> Product2/1
  3x3 Cross Product/1 -> Sum2/3

== system lunar_lander_sim_PWPF_2023a/Subsystem1/Calculate Attitude  ==
  p q r : Inport
  "phi theta psi initial condition " : Inport  Port=2
  " " : Integrator  InitialConditionSource=external
  phidot thetadot psidot : shared6dofsys/DCM & Euler Angles (Euler)/phidot thetadot psidot  SystemSampleTime=-1  VariantActivationTime=update diagram  Latency=0  AutoFrameSizeCalculation=off
  "phi theta psi " : Outport
  phidot thetadot psi : Outport  Port=2
  wires:
  "phi theta psi initial condition "/1 -> " "/2
  " "/1 -> phidot thetadot psidot/2, "phi theta psi "/1
  phidot thetadot psidot/1 -> phidot thetadot psi/1, " "/1
  p q r/1 -> phidot thetadot psidot/1

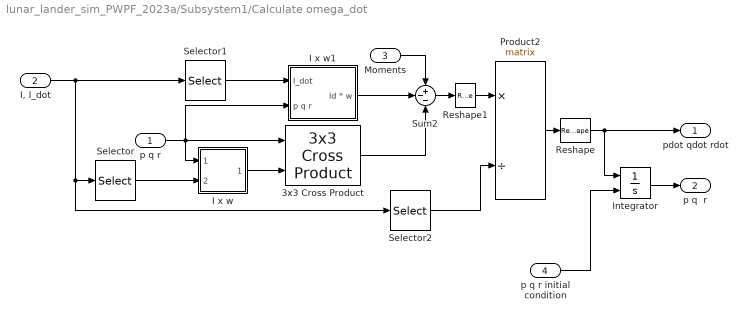
== system lunar_lander_sim_PWPF_2023a/Subsystem1/Calculate omega_dot ==
  p q r : Inport  OutDataTypeStr=double
  "I, I_dot" : Inport  Port=2  OutDataTypeStr=double
  Moments : Inport  Port=3  OutDataTypeStr=double
  p q r initial condition : Inport  Port=4
  3x3 Cross Product : sharedutil/3x3 Cross Product  aMode=aMode
  I x w : Subsystem
  I x w1 : Subsystem
  Integrator : Integrator  InitialConditionSource=external
  Product2 : Product  Inputs=*/  Multiplication=Matrix(*)  SaturateOnIntegerOverflow=on  OutDataTypeStr=Inherit: Same as first input
  Reshape : Reshape
  Reshape1 : Reshape  OutputDimensionality=Row vector (2-D)
  Selector : Selector  NumberOfDimensions=2  InputPortWidth=2  IndexOptions=Index vector (dialog),Select all  Indices=1:3,-1  OutputSizes=1
  Selector1 : Selector  NumberOfDimensions=2  InputPortWidth=2  IndexOptions=Index vector (dialog),Select all  Indices=4:6,-1  OutputSizes=1
  Selector2 : Selector  NumberOfDimensions=2  InputPortWidth=2  IndexOptions=Index vector (dialog),Select all  Indices=1:3,-1  OutputSizes=1
  Sum2 : Sum  Inputs=+--  SaturateOnIntegerOverflow=on
  pdot qdot rdot : Outport  OutDataTypeStr=double  VectorParamsAs1DForOutWhenUnconnected=off
  p q  r : Outport  Port=2
  wires:
  p q r initial condition/1 -> Integrator/2
  Integrator/1 -> p q  r/1
  Reshape/1 -> pdot qdot rdot/1, Integrator/1
  Selector/1 -> I x w/2(Inertia)
  Selector2/1 -> Product2/2
  "I, I_dot"/1 -> Selector/1, Selector2/1, Selector1/1
  p q r/1 -> 3x3 Cross Product/1, I x w1/2(p q r), I x w/1(p q r)
  Product2/1 -> Reshape/1
  Sum2/1 -> Reshape1/1
  Moments/1 -> Sum2/1
  I x w1/1(Id * w) -> Sum2/2
  Selector1/1 -> I x w1/1(I_dot)
  I x w/1(I * w) -> 3x3 Cross Product/2
  Reshape1/1 -> Product2/1
  3x3 Cross Product/1 -> Sum2/3

== system lunar_lander_sim_PWPF_2023a/Subsystem/Calculate omega_dot/I x w ==
  p q r : Inport
  Inertia : Inport  Port=2
  Product : Product  Multiplication=Matrix(*)  InputSameDT=on  SaturateOnIntegerOverflow=on  OutDataTypeStr=Inherit: Same as first input
  Reshape1 : Reshape  OutputDimensionality=Column vector (2-D)
  Reshape2 : Reshape
  I * w : Outport  VectorParamsAs1DForOutWhenUnconnected=off
  wires:
  Product/1 -> Reshape2/1
  Inertia/1 -> Product/1
  p q r/1 -> Reshape1/1
  Reshape1/1 -> Product/2
  Reshape2/1 -> I * w/1

== system lunar_lander_sim_PWPF_2023a/Subsystem/Calculate omega_dot/I x w1 ==
  I_dot : Inport
  p q r : Inport  Port=2
  Product : Product  Multiplication=Matrix(*)  InputSameDT=on  SaturateOnIntegerOverflow=on  OutDataTypeStr=Inherit: Same as first input
  Reshape1 : Reshape  OutputDimensionality=Column vector (2-D)
  Reshape2 : Reshape
  Id * w : Outport  VectorParamsAs1DForOutWhenUnconnected=off
  wires:
  p q r/1 -> Reshape1/1
  I_dot/1 -> Product/1
  Product/1 -> Reshape2/1
  Reshape1/1 -> Product/2
  Reshape2/1 -> Id * w/1

== system lunar_lander_sim_PWPF_2023a/Subsystem1/Calculate omega_dot/I x w ==
  p q r : Inport
  Inertia : Inport  Port=2
  Product : Product  Multiplication=Matrix(*)  InputSameDT=on  SaturateOnIntegerOverflow=on  OutDataTypeStr=Inherit: Same as first input
  Reshape1 : Reshape  OutputDimensionality=Column vector (2-D)
  Reshape2 : Reshape
  I * w : Outport  VectorParamsAs1DForOutWhenUnconnected=off
  wires:
  Product/1 -> Reshape2/1
  Inertia/1 -> Product/1
  p q r/1 -> Reshape1/1
  Reshape1/1 -> Product/2
  Reshape2/1 -> I * w/1

== system lunar_lander_sim_PWPF_2023a/Subsystem1/Calculate omega_dot/I x w1 ==
  I_dot : Inport
  p q r : Inport  Port=2
  Product : Product  Multiplication=Matrix(*)  InputSameDT=on  SaturateOnIntegerOverflow=on  OutDataTypeStr=Inherit: Same as first input
  Reshape1 : Reshape  OutputDimensionality=Column vector (2-D)
  Reshape2 : Reshape
  Id * w : Outport  VectorParamsAs1DForOutWhenUnconnected=off
  wires:
  p q r/1 -> Reshape1/1
  I_dot/1 -> Product/1
  Product/1 -> Reshape2/1
  Reshape1/1 -> Product/2
  Reshape2/1 -> Id * w/1
